simulink model "Projeto_final_psd"  (R2015a)
settings: Solver=FixedStepDiscrete  SolverMode=SingleTasking  StartTime=0.0  StopTime=2  RelTol=1e-3
libraries: dsparch4 x17, dspvision x5, simulink x3, commchan3 x1
settings Model: Creator=aluno  LastModifiedBy=aluno
settings DataIOCC: SignalLoggingSaveFormat=ModelDataLogs  InspectSignalLogs=on
settings OptimizationCC: BlockReduction=off  BooleanDataType=off  ConditionallyExecuteInputs=off  InlineParams=on  ExpressionDepthLimit=2147483647
settings DebuggingCC: AlgebraicLoopMsg=error  SaveWithParameterizedLinksMsg=none  UnderspecifiedInitializationDetection=Classic  MergeDetectMultiDrivingBlocksExec=none  SignalResolutionControl=TryResolveAllWithWarning  MultiTaskDSMMsg=warning  MultiTaskCondExecSysMsg=none  SingleTaskRateTransMsg=error  StateNameClashWarn=warning
settings HardwareCC: ProdHWDeviceType=ASIC/FPGA->ASIC/FPGA  TargetUnknown=on  ProdEqTarget=off

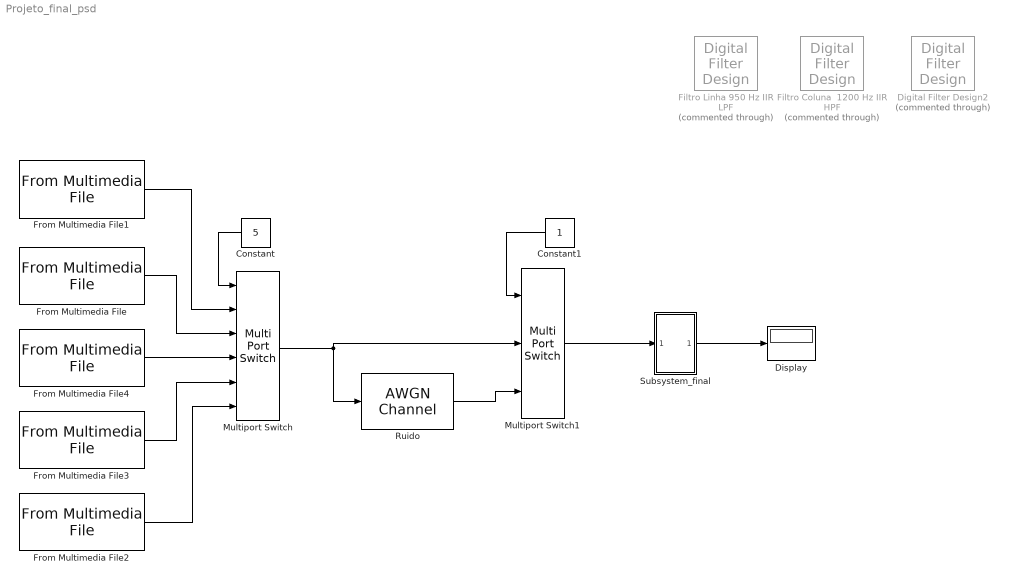
== system Projeto_final_psd ==
  Constant : Constant  Value=5
  Constant1 : Constant
  Digital Filter Design2 : dsparch4/Digital Filter Design  Commented=through  mwdsp_browser_bugfix_var=off
  Display : Display
  Filtro Coluna  1200 Hz IIR HPF : dsparch4/Digital Filter Design  Commented=through  mwdsp_browser_bugfix_var=off
  Filtro Linha 950 Hz IIR LPF : dsparch4/Digital Filter Design  Commented=through  mwdsp_browser_bugfix_var=off
  From Multimedia File : dspvision/From Multimedia File  inputFilename=/home/aluno/Downloads/digito5.wav  loop=on  numPlays=1  outputStreams=Audio only  videoDataType=single  audioDataType=double  inheritSampleTime=on  userDefinedSampleTime=1/30  noAudioOutput=off  isIntensityVideo=off  fourcc=RGB  colorVideoFormat=Separate color signals  outputEOF=off  dataOrg=Column-major  audioFrameSize=1  computeAudioFrameSize=off  outSamplingMode=Sample based
  From Multimedia File1 : dspvision/From Multimedia File  inputFilename=/home/aluno/Downloads/digito4.wav  loop=on  numPlays=1  outputStreams=Audio only  videoDataType=single  audioDataType=double  inheritSampleTime=on  userDefinedSampleTime=1/30  noAudioOutput=off  isIntensityVideo=off  fourcc=RGB  colorVideoFormat=Separate color signals  outputEOF=off  dataOrg=Column-major  audioFrameSize=1  computeAudioFrameSize=off  outSamplingMode=Sample based
  From Multimedia File2 : dspvision/From Multimedia File  inputFilename=/home/aluno/Downloads/todos-digitos1.wav  loop=on  numPlays=1  outputStreams=Audio only  videoDataType=single  audioDataType=double  inheritSampleTime=on  userDefinedSampleTime=1/30  noAudioOutput=off  isIntensityVideo=off  fourcc=RGB  colorVideoFormat=Separate color signals  outputEOF=off  dataOrg=Column-major  audioFrameSize=1  computeAudioFrameSize=off  outSamplingMode=Sample based
  From Multimedia File3 : dspvision/From Multimedia File  inputFilename=/home/aluno/Downloads/digitostar.wav  loop=on  numPlays=1  outputStreams=Audio only  videoDataType=single  audioDataType=double  inheritSampleTime=on  userDefinedSampleTime=1/30  noAudioOutput=off  isIntensityVideo=off  fourcc=RGB  colorVideoFormat=Separate color signals  outputEOF=off  dataOrg=Column-major  audioFrameSize=1  computeAudioFrameSize=off  outSamplingMode=Sample based
  From Multimedia File4 : dspvision/From Multimedia File  inputFilename=/home/aluno/Downloads/digito6.wav  loop=on  numPlays=1  outputStreams=Audio only  videoDataType=single  audioDataType=double  inheritSampleTime=on  userDefinedSampleTime=1/30  noAudioOutput=off  isIntensityVideo=off  fourcc=RGB  colorVideoFormat=Separate color signals  outputEOF=off  dataOrg=Column-major  audioFrameSize=1  computeAudioFrameSize=off  outSamplingMode=Sample based
  Multiport Switch : MultiPortSwitch  Inputs=5
  Multiport Switch1 : MultiPortSwitch  Inputs=2
  "Ruido " : commchan3/AWGN Channel  InputProcessing=Inherited (this choice will be removed - see release notes)  seed=10  noiseMode="Signal to noise ratio  (SNR)"  EbNodB=1  EsNodB=10  SNRdB=60  bitsPerSym=1  Ps=1  Tsym=1  variance=1
  Subsystem_final : Subsystem
  wires:
  From Multimedia File/1 -> Multiport Switch/3
  Multiport Switch/1 -> Multiport Switch1/2, "Ruido "/1
  From Multimedia File1/1 -> Multiport Switch/2
  From Multimedia File4/1 -> Multiport Switch/4
  From Multimedia File3/1 -> Multiport Switch/5
  From Multimedia File2/1 -> Multiport Switch/6
  Constant/1 -> Multiport Switch/1
  "Ruido "/1 -> Multiport Switch1/3
  Multiport Switch1/1 -> Subsystem_final/1(In1)
  Subsystem_final/1(Out1) -> Display/1
  Constant1/1 -> Multiport Switch1/1

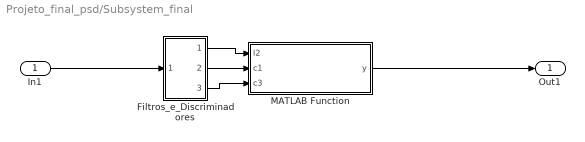
== system Projeto_final_psd/Subsystem_final ==
  In1 : Inport
  Filtros_e_Discriminadores : Subsystem
  MATLAB Function : MATLAB Function  TreatAsAtomicUnit=on
  Out1 : Outport
  wires:
  MATLAB Function/1(y) -> Out1/1
  Filtros_e_Discriminadores/3(Out3) -> MATLAB Function/3(c3)
  Filtros_e_Discriminadores/2(Out2) -> MATLAB Function/2(c1)
  Filtros_e_Discriminadores/1(Out1) -> MATLAB Function/1(l2)
  In1/1 -> Filtros_e_Discriminadores/1(In1)

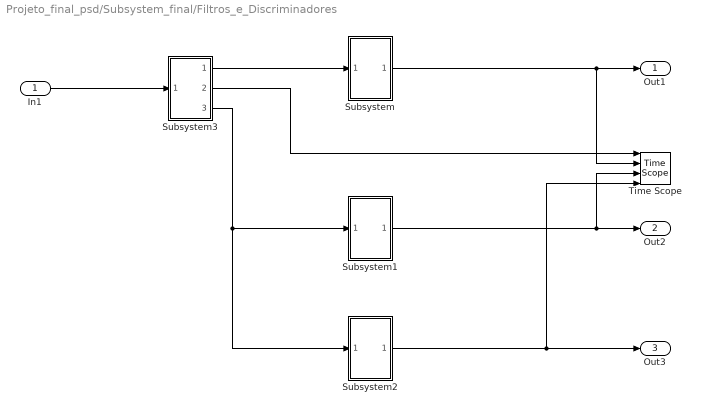
== system Projeto_final_psd/Subsystem_final/Filtros_e_Discriminadores ==
  In1 : Inport
  Subsystem : Subsystem
  Subsystem1 : Subsystem
  Subsystem2 : Subsystem
  Subsystem3 : Subsystem
  Time Scope : TimeScope  DefaultConfigurationName=spbscopes.TimeScopeBlockCfg  NumInputPorts=4
  Out1 : Outport
  Out2 : Outport  Port=2
  Out3 : Outport  Port=3
  wires:
  Subsystem/1(Out1) -> Time Scope/2, Out1/1
  Subsystem1/1(Out1) -> Out2/1, Time Scope/3
  Subsystem2/1(Out1) -> Time Scope/4, Out3/1
  Subsystem3/3(Out3) -> Subsystem2/1(In1), Subsystem1/1(In1)
  In1/1 -> Subsystem3/1(In1)
  Subsystem3/1(Out1) -> Subsystem/1(In1)
  Subsystem3/2(Out2) -> Time Scope/1

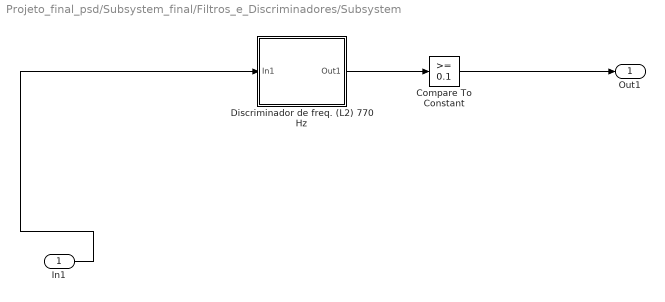
== system Projeto_final_psd/Subsystem_final/Filtros_e_Discriminadores/Subsystem ==
  In1 : Inport
  Compare To Constant : simulink/Logic and Bit Operations/Compare To Constant  relop=>=  const=0.1  OutDataTypeStr=boolean
  Discriminador de freq. (L2) 770 Hz : Subsystem  mask{fp1=0, fc1=0}
  Out1 : Outport
  wires:
  Compare To Constant/1 -> Out1/1
  Discriminador de freq. (L2) 770 Hz/1(Out1) -> Compare To Constant/1
  In1/1 -> Discriminador de freq. (L2) 770 Hz/1(In1)

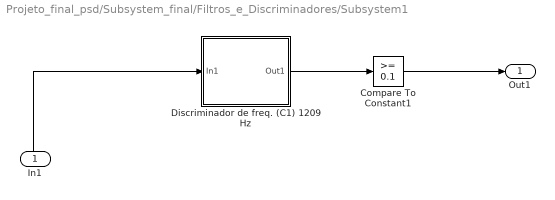
== system Projeto_final_psd/Subsystem_final/Filtros_e_Discriminadores/Subsystem1 ==
  In1 : Inport
  Compare To Constant1 : simulink/Logic and Bit Operations/Compare To Constant  relop=>=  const=0.1  OutDataTypeStr=boolean
  Discriminador de freq. (C1) 1209 Hz : Subsystem  mask{fp1=0, fc1=0}
  Out1 : Outport
  wires:
  In1/1 -> Discriminador de freq. (C1) 1209 Hz/1(In1)
  Compare To Constant1/1 -> Out1/1
  Discriminador de freq. (C1) 1209 Hz/1(Out1) -> Compare To Constant1/1

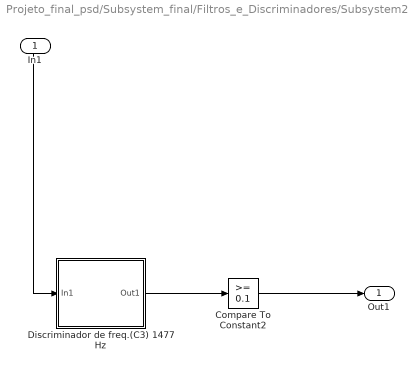
== system Projeto_final_psd/Subsystem_final/Filtros_e_Discriminadores/Subsystem2 ==
  In1 : Inport
  Compare To Constant2 : simulink/Logic and Bit Operations/Compare To Constant  relop=>=  const=0.1  OutDataTypeStr=boolean
  Discriminador de freq.(C3) 1477 Hz : Subsystem
  Out1 : Outport
  wires:
  In1/1 -> Discriminador de freq.(C3) 1477 Hz/1(In1)
  Compare To Constant2/1 -> Out1/1
  Discriminador de freq.(C3) 1477 Hz/1(Out1) -> Compare To Constant2/1

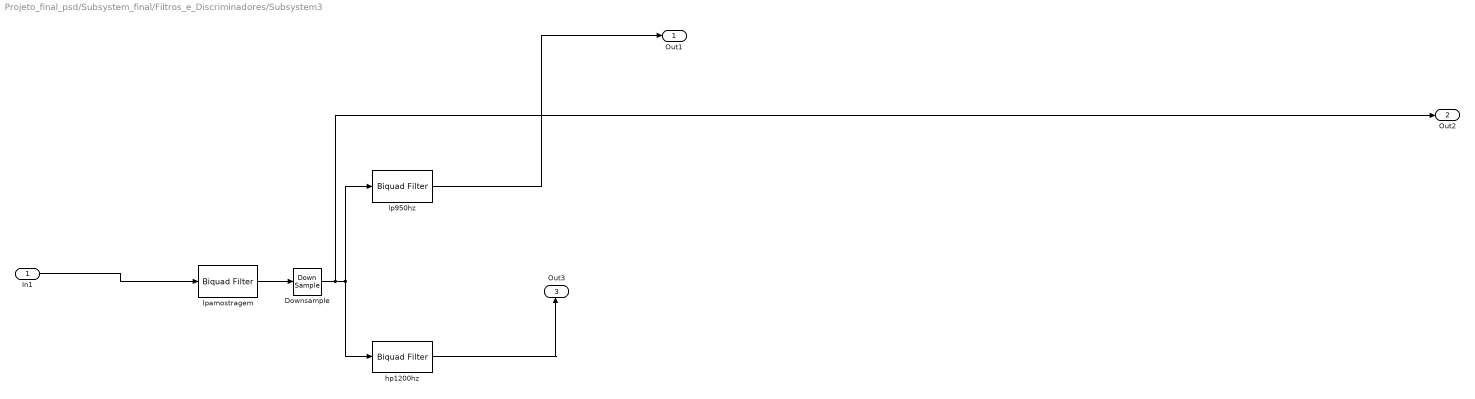
== system Projeto_final_psd/Subsystem_final/Filtros_e_Discriminadores/Subsystem3 ==
  In1 : Inport
  Downsample : DownSample  N=10  phase=1  RateOptions=Allow multirate processing
  hp1200hz : dsparch4/Biquad Filter  Tag=BlockMethodSubSystem  IIRFiltStruct=Direct form II  CoeffSource=Specify via dialog  BiQuadCoeffs=[1 -2 1 1 -1.04350628883651675 0.775318936238440504;1 -2 1 1 -0.859783892439210606 0.462751726222955795;1 -2 1 1 -0.74778917825850344 0.272214937925007283;1 -2 1 1 -0.683137828438767691 0.162223491954589794;1 -2 1 1 -0.653437179328878459 0.11169372960677483]  a0Flag=Warning  IC=0  ICnum=0  ICden=0  denAccumFracLength=30  denProdOutputFracLength=30  secondMemoryFracLength=15  roundingMode=Floor  overflowMode=off  ScaleValues=[0.704706306268739313;0.580633904665541656;0.505001029045877736;0.461340330098339357;0.441282727233913263;1]  optimizeScaleValues=on  ScaleValueMode=Specify via input port (g)  scaleValueFracLength=14  FilterSource=Specify via dialog  FilterObject=Hm_biquad
  lp950hz : dsparch4/Biquad Filter  Tag=BlockMethodSubSystem  IIRFiltStruct=Direct form II  CoeffSource=Specify via dialog  BiQuadCoeffs=[1 2 1 1 -1.32766332900689643 0.808011210261255997;1 2 1 1 -1.12267216099836009 0.528854347473448394;1 2 1 1 -0.992338034266713964 0.351365403505482843;1 2 1 1 -0.915148600767613951 0.246248874313944516;1 2 1 1 -0.879194625152672993 0.197286769580738014]  a0Flag=Warning  IC=0  ICnum=0  ICden=0  denAccumFracLength=30  denProdOutputFracLength=30  secondMemoryFracLength=15  roundingMode=Floor  overflowMode=off  ScaleValues=[0.120086970313589878;0.101545546618772048;0.0897568423096922197;0.0827750683865826065;0.0795230361070162622;1]  optimizeScaleValues=on  ScaleValueMode=Specify via input port (g)  scaleValueFracLength=14  FilterSource=Specify via dialog  FilterObject=Hm_biquad
  lpamostragem : dsparch4/Biquad Filter  Tag=BlockMethodSubSystem  IIRFiltStruct=Direct form II  CoeffSource=Specify via dialog  BiQuadCoeffs=[1 2 1 1 -1.92007944797206209e-16 0.729453817281745076;1 2 1 1 -1.52713931050310268e-16 0.37552480594492188;1 2 1 1 -1.30070718113307607e-16 0.171572875253809959;1 2 1 1 -1.17421384899945951e-16 0.0576378105614484409;1 2 1 1 -1.11709970013985469e-16 0.00619395865710822922]  a0Flag=Warning  IC=0  ICnum=0  ICden=0  denAccumFracLength=30  denProdOutputFracLength=30  secondMemoryFracLength=15  roundingMode=Floor  overflowMode=off  ScaleValues=[0.432363454320436214;0.343881201486230414;0.292893218813452427;0.26440945264036203;0.251548489664277064;1]  optimizeScaleValues=on  ScaleValueMode=Specify via input port (g)  scaleValueFracLength=14  FilterSource=Specify via dialog  FilterObject=Hm_biquad
  Out1 : Outport
  Out2 : Outport  Port=2
  Out3 : Outport  Port=3
  wires:
  lp950hz/1 -> Out1/1
  hp1200hz/1 -> Out3/1
  Downsample/1 -> Out2/1, hp1200hz/1, lp950hz/1
  lpamostragem/1 -> Downsample/1
  In1/1 -> lpamostragem/1

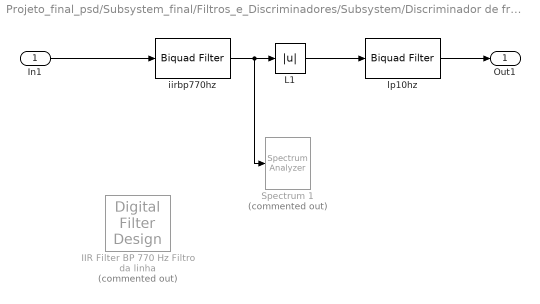
== system Projeto_final_psd/Subsystem_final/Filtros_e_Discriminadores/Subsystem/Discriminador de freq. (L2) 770 Hz ==
  In1 : Inport
  IIR Filter BP 770 Hz Filtro da linha : dsparch4/Digital Filter Design  Commented=on  mwdsp_browser_bugfix_var=off
  L1 : Abs
  Spectrum 1 : SpectrumAnalyzer  Commented=on
  iirbp770hz : dsparch4/Biquad Filter  Tag=BlockMethodSubSystem  IIRFiltStruct=Direct form II  CoeffSource=Specify via dialog  BiQuadCoeffs=[1 0 -1 1 -1.62598721715476158 0.989274264193559461;1 0 -1 1 -1.64706781231817212 0.989555115171887323;1 0 -1 1 -1.62804763549527798 0.978939048381491372]  a0Flag=Warning  IC=0  ICnum=0  ICden=0  denAccumFracLength=30  denProdOutputFracLength=30  secondMemoryFracLength=15  roundingMode=Floor  overflowMode=off  ScaleValues=[0.0105857698857168784;0.0105857698857168784;0.0105304758092542861;1]  optimizeScaleValues=on  ScaleValueMode=Specify via input port (g)  scaleValueFracLength=14  FilterSource=Specify via dialog  FilterObject=Hm_biquad
  lp10hz : dsparch4/Biquad Filter  Tag=BlockMethodSubSystem  IIRFiltStruct=Direct form II  CoeffSource=Specify via dialog  BiQuadCoeffs=[1 2 1 1 -1.99394539724870445 0.99400689711771717;1 2 1 1 -1.98553118528947725 0.985592425636371616]  a0Flag=Warning  IC=0  ICnum=0  ICden=0  denAccumFracLength=30  denProdOutputFracLength=30  secondMemoryFracLength=15  roundingMode=Floor  overflowMode=off  ScaleValues=[1.53749672531671068e-05;1.5310086723583485e-05;1]  optimizeScaleValues=on  ScaleValueMode=Specify via input port (g)  scaleValueFracLength=14  FilterSource=Specify via dialog  FilterObject=Hm_biquad
  Out1 : Outport
  wires:
  L1/1 -> lp10hz/1
  lp10hz/1 -> Out1/1
  In1/1 -> iirbp770hz/1
  iirbp770hz/1 -> Spectrum 1/1, L1/1

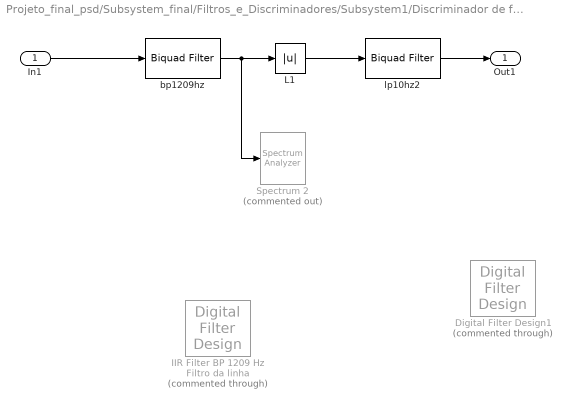
== system Projeto_final_psd/Subsystem_final/Filtros_e_Discriminadores/Subsystem1/Discriminador de freq. (C1) 1209 Hz ==
  In1 : Inport
  Digital Filter Design1 : dsparch4/Digital Filter Design  Commented=through  mwdsp_browser_bugfix_var=off
  IIR Filter BP 1209 Hz Filtro da linha : dsparch4/Digital Filter Design  Commented=through  mwdsp_browser_bugfix_var=off
  L1 : Abs
  Spectrum 2 : SpectrumAnalyzer  Commented=on
  bp1209hz : dsparch4/Biquad Filter  Tag=BlockMethodSubSystem  IIRFiltStruct=Direct form II  CoeffSource=Specify via dialog  BiQuadCoeffs=[1 0 -1 1 -1.13271476640616209 0.984159087873017979;1 0 -1 1 -1.17708939331535545 0.984464316839553266;1 0 -1 1 -1.14612330330778067 0.968861838847255963]  a0Flag=Warning  IC=0  ICnum=0  ICden=0  InputProcessing=Columns as channels (frame based)  denAccumFracLength=30  denProdOutputFracLength=30  secondMemoryFracLength=15  roundingMode=Floor  overflowMode=off  ScaleValues=[0.0156897810066821304;0.0156897810066821304;0.0155690805763720515;1]  optimizeScaleValues=on  ScaleValueMode=Specify via input port (g)  scaleValueFracLength=14  FilterSource=Specify via dialog  FilterObject=Hm_biquad
  lp10hz2 : dsparch4/Biquad Filter  Tag=BlockMethodSubSystem  IIRFiltStruct=Direct form II  CoeffSource=Specify via dialog  BiQuadCoeffs=[1 2 1 1 -1.99394539724870445 0.99400689711771717;1 2 1 1 -1.98553118528947725 0.985592425636371616]  a0Flag=Warning  IC=0  ICnum=0  ICden=0  InputProcessing=Columns as channels (frame based)  denAccumFracLength=30  denProdOutputFracLength=30  secondMemoryFracLength=15  roundingMode=Floor  overflowMode=off  ScaleValues=[1.53749672531671068e-05;1.5310086723583485e-05;1]  optimizeScaleValues=on  ScaleValueMode=Specify via input port (g)  scaleValueFracLength=14  FilterSource=Specify via dialog  FilterObject=Hm_biquad
  Out1 : Outport
  wires:
  L1/1 -> lp10hz2/1
  lp10hz2/1 -> Out1/1
  In1/1 -> bp1209hz/1
  bp1209hz/1 -> Spectrum 2/1, L1/1

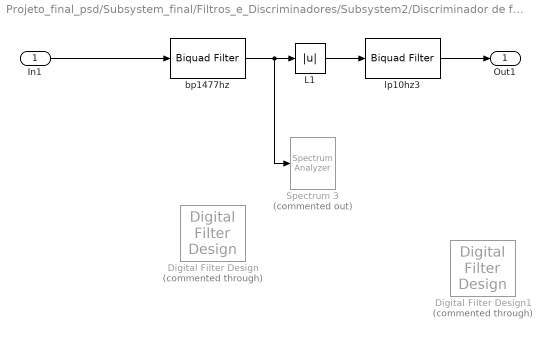
== system Projeto_final_psd/Subsystem_final/Filtros_e_Discriminadores/Subsystem2/Discriminador de freq.(C3) 1477 Hz ==
  In1 : Inport
  Digital Filter Design : dsparch4/Digital Filter Design  Commented=through  mwdsp_browser_bugfix_var=off
  Digital Filter Design1 : dsparch4/Digital Filter Design  Commented=through  mwdsp_browser_bugfix_var=off
  L1 : Abs
  Spectrum 3 : SpectrumAnalyzer  Commented=on
  bp1477hz : dsparch4/Biquad Filter  Tag=BlockMethodSubSystem  IIRFiltStruct=Direct form II  CoeffSource=Specify via dialog  BiQuadCoeffs=[1 0 -1 1 -0.820943011203163486 0.981342997812801654;1 0 -1 1 -0.761149127706174378 0.981076547755722173;1 0 -1 1 -0.783888954994804932 0.962759448275491092]  a0Flag=Warning  IC=0  ICnum=0  ICden=0  InputProcessing=Columns as channels (frame based)  denAccumFracLength=30  denProdOutputFracLength=30  secondMemoryFracLength=15  roundingMode=Floor  overflowMode=off  ScaleValues=[0.0187927729731211524;0.0187927729731211524;0.0186202758622544193;1]  optimizeScaleValues=on  ScaleValueMode=Specify via input port (g)  scaleValueFracLength=14  FilterSource=Specify via dialog  FilterObject=Hm_biquad
  lp10hz3 : dsparch4/Biquad Filter  Tag=BlockMethodSubSystem  IIRFiltStruct=Direct form II  CoeffSource=Specify via dialog  BiQuadCoeffs=[1 2 1 1 -1.99588120945958036 0.995942769035442321;1 2 1 1 -1.98889290589965295 0.988954249933126528;1 2 1 1 -1.98488044514143502 0.984941665417351508]  a0Flag=Warning  IC=0  ICnum=0  ICden=0  InputProcessing=Columns as channels (frame based)  denAccumFracLength=30  denProdOutputFracLength=30  secondMemoryFracLength=15  roundingMode=Floor  overflowMode=off  ScaleValues=[1.53898939654991318e-05;1.53360083683622574e-05;1.53050689791255494e-05;1]  optimizeScaleValues=on  ScaleValueMode=Specify via input port (g)  scaleValueFracLength=14  FilterSource=Specify via dialog  FilterObject=Hm_biquad
  Out1 : Outport
  wires:
  L1/1 -> lp10hz3/1
  lp10hz3/1 -> Out1/1
  In1/1 -> bp1477hz/1
  bp1477hz/1 -> Spectrum 3/1, L1/1

== matlab function Projeto_final_psd/Subsystem_final/MATLAB Function ==
  data: l2 input; y output; c1 input; c3 input
function y = detector_de_tecla(l2, c1, c3)

%deteccao dos caracteres 4, 6, 5 e *. Como smente possuimos 1 linha e 2
%colunas, nao ha condicoes suficientes para detectar os digitos 5 e *, logo
%sera erro

u = '';
    if((l2 == 1) && (c1 == 1) && (c3 == 0) )
        u = 4;
    
    elseif((l2 == 1) && (c1 == 0) && (c3 == 1))
        u = 6;
    
    else 
        u = 14;  %14 significa E em ascii conversao decimal, de erro
    end; 
   
y = u;
